simulink model "RLS2_5_NS"  (R2024a)
settings: Solver=FixedStepAuto  StartTime=0.0  StopTime=500  FixedStep=0.3  RelTol=1e-3
libraries: simulink x2, dspsrcs4 x2, cstblocks x1
settings Model: Creator=mergenelos  LastModifiedBy=mergenelos

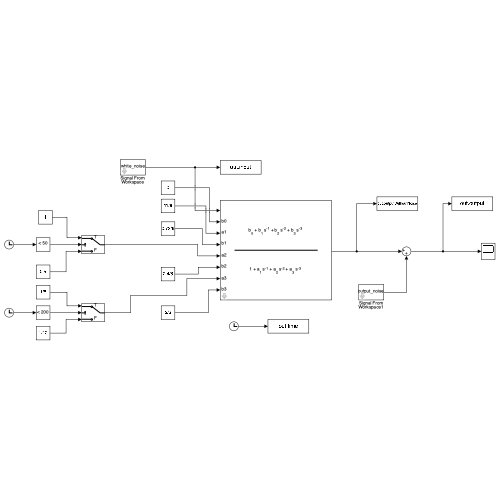
[thumbnail: Simulink's stored preview of the top-level diagram]
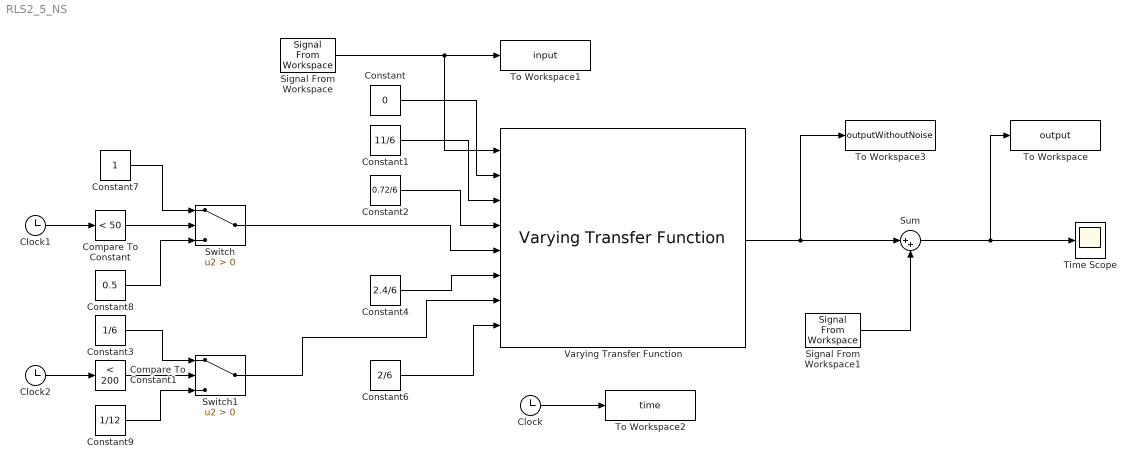
== system RLS2_5_NS ==
  Clock : Clock
  Clock1 : Clock
  Clock2 : Clock
  Compare To Constant : simulink/Logic and Bit Operations/Compare To Constant  relop=<  const=50  OutDataTypeStr=boolean
  Compare To Constant1 : simulink/Logic and Bit Operations/Compare To Constant  relop=<  const=200  OutDataTypeStr=boolean
  Constant : Constant  Value=0
  Constant1 : Constant  Value=11/6
  Constant2 : Constant  Value=0.72/6
  Constant3 : Constant  Value=1/6
  Constant4 : Constant  Value=2.4/6
  Constant6 : Constant  Value=2/6
  Constant7 : Constant
  Constant8 : Constant  Value=0.5
  Constant9 : Constant  Value=1/12
  Signal From Workspace : dspsrcs4/Signal From Workspace  X=white_noise  Ts=0.3  nsamps=1  OutputAfterFinalValue=Setting to zero  ignoreOrWarnInputAndFrameLengths=off  OutputFrames=off
  Signal From Workspace1 : dspsrcs4/Signal From Workspace  X=output_noise  Ts=0.3  nsamps=1  OutputAfterFinalValue=Setting to zero  ignoreOrWarnInputAndFrameLengths=off  OutputFrames=off
  Sum : Sum  Inputs=|++
  Switch : Switch  Criteria=u2 > Threshold  SaturateOnIntegerOverflow=off  InputSameDT=off
  Switch1 : Switch  Criteria=u2 > Threshold  SaturateOnIntegerOverflow=off  InputSameDT=off
  Time Scope : Scope
  To Workspace : ToWorkspace  VariableName=output  SaveFormat=Timeseries  SampleTime=-1
  To Workspace1 : ToWorkspace  VariableName=input  SaveFormat=Timeseries  SampleTime=-1
  To Workspace2 : ToWorkspace  VariableName=time  SaveFormat=Timeseries  SampleTime=-1
  To Workspace3 : ToWorkspace  VariableName=outputWithoutNoise  SaveFormat=Timeseries  SampleTime=-1
  Varying Transfer Function : cstblocks/Linear Parameter Varying/Varying Transfer Function  N=3  Feedthrough=on
  wires:
  Signal From Workspace/1 -> To Workspace1/1, Varying Transfer Function/1
  Clock/1 -> To Workspace2/1
  Sum/1 -> Time Scope/1, To Workspace/1
  Signal From Workspace1/1 -> Sum/2
  Constant/1 -> Varying Transfer Function/2
  Constant1/1 -> Varying Transfer Function/3
  Constant2/1 -> Varying Transfer Function/4
  Constant4/1 -> Varying Transfer Function/6
  Constant6/1 -> Varying Transfer Function/8
  Varying Transfer Function/1 -> To Workspace3/1, Sum/1
  Switch/1 -> Varying Transfer Function/5
  Constant7/1 -> Switch/1
  Clock1/1 -> Compare To Constant/1
  Compare To Constant/1 -> Switch/2
  Constant8/1 -> Switch/3
  Compare To Constant1/1 -> Switch1/2
  Clock2/1 -> Compare To Constant1/1
  Constant9/1 -> Switch1/3
  Constant3/1 -> Switch1/1
  Switch1/1 -> Varying Transfer Function/7
